simulink model "sensorMCU"  (Simulink 6.6)
settings: Solver=FixedStepDiscrete  StartTime=0.0  StopTime=10.0  FixedStep=0.01  RelTol=1e-3
InitFcn:
  | mcuInit
values from neighbouring files (symbols this model uses):
  gxGainrad = gxGain*pi/180    [mcuInit.m]
  gyGainrad = gyGain*pi/180    [mcuInit.m]
  gzGainrad = gzGain*pi/180    [mcuInit.m]
  T = 0.01    [initGPS.m]    (also in mcuInit.m)
undefined symbols (not defined in the file or in its folder): AccelParam, floatToBytes, gaind, gpsInit, gpsParse, gpsRead, gpsSeparate, gyTGain, hil_getEuler, hil_getGPSRead, hil_getRates, hil_getRawRead, hil_getVned, hil_getXYZ, hilRead, logData, loggerInit, MagParam, mzTGain, polesd, protParseDecode, protParserInit, shortToBytes, spiMasterInit, spiSend, stTGain, tmeanMz, tmeanSt, tmeanVl, u1, uartInit, uShortToBytes, vlTGain, y1, zerosd
libraries: dsPICdrivers x72, simulink x6, dspswit3 x1, dspsigops x1, xpclib x1, aerolibconvert2 x1
(part 3 of 3)

== matlab function Position-Attitude Filter/kalman filter ==
  data: bias_out output inherited; quatout output inherited; V_inertial_out output inherited; w input inherited; acc input inherited; mags input inherited; windV input inherited; dt_gps input inherited; gps_update input inherited; XY_inertial input inherited; baro input inherited; gps_psi input inherited; euler_out output inherited; pqr_out output inherited; unfiltered_euler_out output inherited; bodyAcc_out output inherited; P_out output inherited
function [bias_out, quatout,V_inertial_out,euler_out,pqr_out,unfiltered_euler_out,bodyAcc_out,P_out] = fcn(w,acc,mags,windV,dt_gps,gps_update,XY_inertial,baro,gps_psi)

    %% initialize static variables
    persistent xhat;
    persistent P;
    persistent bodyV_prev;
	persistent XY_inertial_prev;
    persistent baro_prev;
    persistent unfiltered_euler;
    persistent bodyAcc;
    persistent V_inertial;
	persistent qerr;
    persistent gps_alive;
    if isempty(xhat)
        xhat = [0.999998858349755;
                0.000871902307597;
                0.000873425393729;
                0.000871902307597;
                w+[.001;.001;.001]];
        P=diag( [ 1*ones(1,3) .05*ones(1,3) ] );
        bodyV_prev = [0;0;0];
        baro_prev = baro;
        XY_inertial_prev = [0;0];
        unfiltered_euler = [0;0;0];
        bodyAcc = [0;0;0];
        V_inertial = [0;0;0];
        qerr = [1;0;0;0];
        gps_alive = 0;
    end

    %% initialize other variables
    dt  = 0.01;      % fundamental time step
    
    B = [0.468741473405951;
         0.129010679377825;
        -0.873863648240210];
    
    Yaw_good_threshold = 6; %if GPS interpolated velocity is greater than 8, use GPS heading
    dt_gps_thresh= 2;

    H= [eye(3,3) zeros(3,3)]; % measurement matrix
    F= zeros(6,6);				% State transition matrix
    Gw=zeros(6,6);				% Noise mapping matrix
    Rw=eye(6,6);					% Process noise covariance

    % kalman filter parameters
    rwt = .02;       % error quaternion noise
    rwb = 1e-3;       % gyro bias noise
    % rwb = 0.01;
    rvv = .04;        % sensor noise
    % rvv = 0.25;

    F(1:3,4:6) = 0.5*eye(3);		% the state transition matrix
    
%     Gw(1:3,1:3) = -0.5*eye(3);	% Process Noise input
%     Gw(4:6,4:6) = eye(3);			% Process Noise input
%     Rw(1:3,1:3) = rwt^2*eye(3);	% Covariance of process noise
%     Rw(4:6,4:6) = rwb^2*eye(3);	% Covariance of process noise
%     Cd=dt*Gw*Rw*transpose(Gw);  % discreet equivalent of noise
    Cd = [diag(dt*.25*rwt^2*ones(3,1)),                   zeros(3,3);
                            zeros(3,3), diag(dt*.25*rwb^2*ones(3,1));];

	Rv = rvv^2*eye(3);			% measurement noise covariance
    
    %% integrate gyros to get new xhat
    xhat(1:4) = integ_gyros(xhat,w,dt);
    
    %% fill in the state transition matrix, Phi = expm(F*dt)
    Phi = state_transition(xhat,w,dt);
    
    %% propogate covariance: P=Phi*(P+Cd)*transpose(Phi);
    for k=1:6
        P(k,k)=P(k,k)+Cd(k,k);  % P = P+Cd
    end
    %% P=Phi*P*transpose(Phi);
    P(1:3,:)=[(Phi(1:3,1:3)*P(1:3,:)+Phi(1:3,4:6)*P(4:6,:))*transpose(Phi(1:3,:))  Phi(1:3,:)*P(:,4:6)];
    P(4:6,:)=[transpose(P(1:3,4:6)) P(4:6,4:6);];


    %% check for gps update
    if (gps_alive == 0)
        body = [0;0;0];
        [Pitch, Roll, Yaw] = accelMagsBody2euler(acc,mags,body);


        % %         q_hat = xhat(1:4);
% %         for k=1
% %             Cnb = q2dcm(q_hat);
% %             A_i = transpose(Cnb)*Gbody;
% %             B_i = transpose(Cnb)*mags;
% %             M = -[2*sk([0;0;-1]);2*sk(B)];
% %             qerr = inv(M'*M)*M'*-([A_i-[0;0;-1];B_i-B]);
% % 
% %             if norm(qerr)^2 < 1
% %                 q_hat=quatmult([sqrt(1-norm(qerr)^2);qerr],q_hat);
% %             else
% %                 q_hat=quatmult([1;qerr],q_hat);
% %             end
% %             if (q_hat(1)<0)
% %                 q_hat = -q_hat;            					% make scalar part positive
% %             end
% %           q_hat=q_hat/norm(q_hat);
% %         end

        unfiltered_euler = [Roll; Pitch; Yaw]*57.2958;
        

        
        %
        % Now use the euler angles from GPS/Acc to compute the measured quaternion
        %
        qhat = xhat(1:4);						% pull out qhat from state
        bhat = xhat(5:7);						% pull out gyro bias estimates
        qm = eul2quat([Roll Pitch Yaw]);			% measurement quaternion
        if (qm(1)<0)
            qm = -qm;            					% make scalar part positive
        end
        qerr = quatmult(quatinv(qhat),qm);			% formulate error quaternion
        if qerr(1)<0
            qerr=-qerr;
        end
%        L = P*H'*inv(H*P*H' + Rv);					% compute gains
        HPHpR = P(1:3,1:3);
        for k=1:3
            HPHpR(k,k)=HPHpR(k,k)+Rv(k,k);
        end
        invHPHpR = inv(HPHpR);
        L = P(:,1:3)*invHPHpR;					% compute gains
%        P = (eye(6) - [L zeros(6,3)])*P;						% update covariance matrix
        Mtemp = -L(1:3,:);
        for k=1:3
            Mtemp(k,k)=Mtemp(k,k)+1;
        end
        P = [                          Mtemp*P(1:3,1:3),               Mtemp*P(1:3,4:6);
             -L(4:6,:)*P(1:3,1:3)+transpose(P(1:3,4:6)),-L(4:6,:)*P(1:3,4:6)+P(4:6,4:6);];
        ds = L*qerr(2:4);								% generate updates
 %       ds = L*qerr;								% generate updates
        qhat_plus = quatmult(qhat,[1;ds(1:3)]);	% generate new attitude estimate
        bhat_plus = bhat - ds(4:6);					% generate the new gyro biases
        qhat_plus = qhat_plus/norm(qhat_plus);		% renormalize quaternion
        if (qhat_plus(1)<0)
            qhat_plus = -qhat_plus;					% make scalar part positive
        end
        xhat(1:4) = qhat_plus;				% put attitude estimate back into state
        xhat(5:7) = bhat_plus;				% put gyro bias estimates back into state

    else
%         if (gps_update)									% gps update recieved
%             if (dt_gps < dt_gps_thresh)
%                 gps_alive = 1;
%             end
%             V_inertial = ([XY_inertial-XY_inertial_prev;baro-baro_prev])/dt_gps;
%             XY_inertial_prev=XY_inertial;
%             baro_prev = baro;
%    
%             if (  (norm(V_inertial(1:2))>Yaw_good_threshold) && (gps_alive)  )
%                 Yaw = gps_psi;
%             else
%                 Yaw = quat2psi(xhat(1:4));
%             end
% 
%             Cnb = q2dcm(xhat(1:4));
%             %   aircraftV =V_inertial - windV; 				% V_gps = V_aircraft + V_wind
% 
%             bodyV=Cnb*V_inertial;
%             bodyAcc = (bodyV - bodyV_prev)/dt_gps;	% generate the body acceleration
%             if (bodyV_prev(1) == 0 && bodyV_prev(2) == 0)
%                  bodyAcc = [0;0;0];
%             end
%             bodyV_prev = bodyV;							% store body velocity for next step
% 
%             % if GPS update comes in reasonable time, use body accel, else don't
%             if gps_alive
%                  Gbody = acc - bodyAcc;
%             else
%                 Gbody = acc;
%             end
%             Gbody = Gbody/norm(Gbody)*.99999999;
%             Pitch = asin(Gbody(1));
%             Roll = asin(-Gbody(2)/cos(Pitch));
%             if sign(Gbody(3)) >= 0   % if upside down, correct phi
%                 Roll=-Roll-pi*sign(Gbody(2));
%             end
%             unfiltered_euler = [Roll; Pitch; Yaw];
%    
%             %
%             % Now use the euler angles from GPS/Acc to compute the measured quaternion
%             %
%             qhat = xhat(1:4);						% pull out qhat from state
%             bhat = xhat(5:7);						% pull out gyro bias estimates
%             qm = eul2quat([Roll Pitch Yaw]);			% measurement quaternion
%             if (qm(1)<0)
%                 qm = -qm;            					% make scalar part positive
%             end
%             qerr = quatmult(quatinv(qhat),qm);			% formulate error quaternion
%             L = P*H'*inv(H*P*H' + Rv);					% compute gains
%             P = (eye(6) - L*H)*P;						% update covariance matrix
%             ds = L*qerr(2:4);								% generate updates
%             qhat_plus = quatmult(qhat,[1;ds(1:3)]);	% generate new attitude estimate
%             bhat_plus = bhat - ds(4:6);					% generate the new gyro biases
%             qhat_plus = qhat_plus/norm(qhat_plus);		% renormalize quaternion
%             if (qhat_plus(1)<0)
%                 qhat_plus = -qhat_plus;					% make scalar part positive
%             end
%             xhat(1:4) = qhat_plus;				% put attitude estimate back into state
%             xhat(5:7) = bhat_plus;				% put gyro bias estimates back into state
%         end
    end

    
    
    P_out = P;
    quatout = xhat(1:4);
    euler_out = quat2eul(quatout);
%     euler_out = mags*pi/180;
%     euler_out = unfiltered_euler;
    euler_out(1) = -euler_out(1);
    bias_out = xhat(5:7);
    pqr_out = [w(1)-xhat(5);
               w(2)-xhat(6);
               w(3)-xhat(7);];
    unfiltered_euler_out = unfiltered_euler;
    bodyAcc_out = bodyAcc;
    V_inertial_out = V_inertial;
    
end






%================================================================
%==================   additional functions ======================
%================================================================
function quat = integ_gyros(xhat,w,dt)
    p  = w(1) - xhat(5);
    q  = w(2) - xhat(6);
    r  = w(3) - xhat(7);
    normomega    = norm([p;q;r]);
    normomegainv = inv(normomega);
    C  = cos(.5*dt*normomega);
    Sn = sin(.5*dt*normomega)*normomegainv;

    Phi_old_small = [    C, -(p *Sn), -(q* Sn), -(r *Sn);
                   (p *Sn),        C,  (r* Sn), -(q *Sn);
                   (q* Sn), -(r *Sn),        C,  (p* Sn);
                   (r* Sn),  (q *Sn), -(p* Sn),        C;];
    xhat(1:4) = Phi_old_small*xhat(1:4);	       % insert back into state
    if xhat(1)<0
        xhat(1:4)=-xhat(1:4);
    end
    quat = xhat(1:4)/norm(xhat(1:4));  %normalize quaternion
end

function Phi = state_transition(xhat,w,dt)
    p  = w(1) - xhat(5);
    q  = w(2) - xhat(6);
    r  = w(3) - xhat(7);
    p2 = p*p;
    q2 = q*q;
    r2 = r*r;
    pq = p*q;
    pr = p*r;
    qr = q*r;
    omega = sqrt(p2+q2+r2);
    omega2 = omega*omega;
    omega3 = omega2*omega;
    omega2inv = inv(omega2);
    omega3inv = inv(omega3);
    cdo = cos(dt*omega);
    sdo = sin(dt*omega);
    Phi = [       (p2 + cdo*(q2 + r2))*omega2inv, (pq - cdo*pq + omega*r*sdo)*omega2inv, (pr - cdo*pr - omega*q*sdo)*omega2inv,                 (dt*omega*p2 + (q2 + r2)*sdo)*.5*omega3inv, -(-dt*omega*pq + (-1 + cdo)*omega*r + pq*sdo)*.5*omega3inv, (dt*omega*pr + (-1 + cdo)*omega*q - pr*sdo)*.5*omega3inv;
           (pq - cdo*pq - omega*r*sdo)*omega2inv,        (q2 + cdo*(p2 + r2))*omega2inv, (qr - cdo*qr + omega*p*sdo)*omega2inv,   (dt*omega*pq + (-1 + cdo)*omega*r - pq*sdo)*.5*omega3inv,                 (dt*omega*q2 + (p2 + r2)*sdo)*.5*omega3inv,        (omega*(p - cdo*p + dt*qr) - qr*sdo)*.5*omega3inv;
           (pr - cdo*pr + omega*q*sdo)*omega2inv, (qr - cdo*qr - omega*p*sdo)*omega2inv,        (cdo*(p2 + q2) + r2)*omega2inv, -(-dt*omega*pr + (-1 + cdo)*omega*q + pr*sdo)*.5*omega3inv,       (omega*((-1 + cdo)*p + dt*qr) - qr*sdo)*.5*omega3inv,               (dt*omega*r2 + (p2 + q2)*sdo)*.5*omega3inv;
           0, 0, 0, 1, 0, 0;
           0, 0, 0, 0, 1, 0;
           0, 0, 0, 0, 0, 1];
end


function [Pitch, Roll, Yaw] = accelMagsBody2euler(acc,mags,body)
    Gbody = acc-body;
    Gbody = Gbody/norm(Gbody)*.99999999;
    Pitch = asin(Gbody(1));
    temp = -Gbody(2)/cos(Pitch);
	if abs(temp)<1
    	Roll = asin(-Gbody(2)/cos(Pitch));
	else
    	Roll = pi/2*sign(temp);
    end
        
	if sign(Gbody(3)) >= 0   % if upside down, correct phi
        Roll=-Roll-pi*sign(Gbody(2));
    end

    ct = cos(Pitch); %set up trig for less computation time
    st = sin(Pitch);
    cp = cos(Roll);
    sp = sin(Roll);
    Bflat = [ct, st*sp, cp*st;
              0,    cp,   -sp;]*mags; %rotate mags into phi=0, theta=0
	Yaw = 0.2686 -atan2g(Bflat(2),Bflat(1)); %calculate psi
end


function as=sk(a)
    % This function determines the skew-symmetric matrix
    % corresponding to a given vector a with three elements.
    	as=[0 -a(3) a(2); a(3) 0 -a(1); -a(2) a(1) 0];
end


function quat = quatmult(q1,q2)
    %   Multiplies two quaternions.
    qv1 = q1(2:4);
    qs1 = q1(1);
    qv2 = q2(2:4);
    qs2 = q2(1);

    quatv = cross(qv1,qv2) + qs1*qv2 + qs2*qv1;
    quats = qs1*qs2 - dot(qv1,qv2);

    quat = [quats;quatv];
end


function quat = quatinv(q)
    %   Inverts a quaternion.
    quat = [q(1);-q(2:4)];
end


function angles = quat2eul( q )
    qin = q./norm(q);

    y=2.*(qin(3,1).*qin(4,1) + qin(1,1).*qin(2,1));
    x=qin(1,1).^2 - qin(2,1).^2 - qin(3,1).^2 + qin(4,1).^2;
    phi = atan2g(y,x);

    theta = asin(-2.*(qin(2,1).*qin(4,1) - qin(1,1).*qin(3,1)));

    y=2.*(qin(2,1).*qin(3,1) + qin(1,1).*qin(4,1));
    x=qin(1,1).^2 + qin(2,1).^2 - qin(3,1).^2 - qin(4,1).^2;
    psi = atan2g(y,x);

    angles = [phi; theta; psi];
end


function angle = atan2g(y,x)
    angle = 0.;
    if x>0
        angle = atan(y/x);
    end
    if x==0
        angle = .5*pi*sign(y);
    end
    if x<0
        angle = pi*sign(y)+atan(y/x);
    end
end

function q = eul2quat(angles)
    % converts phi,theta,phi into q
    % lifted straight from matlab's function (with a transposed output):
    cang = cos( angles/2 );
    sang = sin( angles/2 );

    q = [ cang(:,1).*cang(:,2).*cang(:,3) + sang(:,1).*sang(:,2).*sang(:,3);
           sang(:,1).*cang(:,2).*cang(:,3) - cang(:,1).*sang(:,2).*sang(:,3);
           cang(:,1).*sang(:,2).*cang(:,3) + sang(:,1).*cang(:,2).*sang(:,3);
           cang(:,1).*cang(:,2).*sang(:,3) - sang(:,1).*sang(:,2).*cang(:,3)];
end

function dcm = q2dcm( q )
    %   The direction cosine matrix performs the coordinate
    %   transformation of a vector in inertial axes to a vector in body axes.

    qin = q; % don't need to normalize because it is already done
    %qin = quatnormalize( q );

    dcm = zeros(3,3);

    dcm(1,1) = qin(1).^2 + qin(2).^2 - qin(3).^2 - qin(4).^2;
    dcm(1,2) = 2.*(qin(2).*qin(3) + qin(1).*qin(4));
    dcm(1,3) = 2.*(qin(2).*qin(4) - qin(1).*qin(3));
    dcm(2,1) = 2.*(qin(2).*qin(3) - qin(1).*qin(4));
    dcm(2,2) = qin(1).^2 - qin(2).^2 + qin(3).^2 - qin(4).^2;
    dcm(2,3) = 2.*(qin(3).*qin(4) + qin(1).*qin(2));
    dcm(3,1) = 2.*(qin(2).*qin(4) + qin(1).*qin(3));
    dcm(3,2) = 2.*(qin(3).*qin(4) - qin(1).*qin(2));
    dcm(3,3) = qin(1).^2 - qin(2).^2 - qin(3).^2 + qin(4).^2;
end



% function Cd=disrw(F,G,Ts,Rwpsd)
% %----------------------------------------------------------------
% %   function [Cd]=disrw(F,G,T,Rwpsd)
% %
% %   disrw computes the discrete equivalent of continous noise for the
% %   dynamic system described by
% %
% %                            x_dot = Fx + Gw
% %
% %   w is the driving noise.  Ts is the sampling time and Rwpsd
% %   is the power spectral density of the driving noise.
% %
% %---------------------------------------------------------------------
% 
% ZF=zeros(size(F));
% [n,m]=size(G);
% ME=[-F G*Rwpsd*G';
%     ZF F'];
% phi=expm(ME*Ts);
% phi12=phi(1:n,n+1:2*n);
% phi22=phi(n+1:2*n,n+1:2*n);
% Cd=phi22'*phi12;
% 
% end

== matlab function myMux Fun4 ==
  data: u1 input inherited; y output inherited; u2 input inherited
function y = myMux(u1, u2)
% This block supports an embeddable subset of the MATLAB language.
% See the help menu for details. 

y = [u1(1:12); u2(1:12)];

== matlab function myMux Fun1 ==
  data: u1 input inherited; y output inherited; u2 input inherited; u3 input inherited
function y = myMux(u1, u2, u3)
% This block supports an embeddable subset of the MATLAB language.
% See the help menu for details. 

y = zeros(3,1);
y(1) = u1(1);
y(2) = u2(1);
y(3) = u3(1);

== matlab function Position-Attitude Filter/myMux Fun4 ==
  data: u1 input inherited; y output inherited; u2 input inherited
function y = myMux(u1, u2)
% This block supports an embeddable subset of the MATLAB language.
% See the help menu for details. 

y = [u1(1:2); u2];

== matlab function Sensor Data/Raw Sensors/Sensor Suite/myMux Fun3 ==
  data: u1 input inherited; y output inherited; u2 input inherited; u3 input inherited
function y = myMux(u1, u2, u3)
% This block supports an embeddable subset of the MATLAB language.
% See the help menu for details. 

y = [u1(1); u2(1); u3(1)];

== matlab function Sensor Data/Raw Sensors/Sensor Suite/Calibration and Temperature Compensation/Enables/Disables the Computation of initial Biases and Temps ==
  data: tOut output inherited
function tOut = getTIni

persistent aveCount;
persistent tIni;

if isempty(aveCount)
    aveCount =1;
    tIni = 1;
end;

if aveCount < 500
    aveCount = aveCount + 1;
end

if aveCount == 500
    tIni =0;
    aveCount = aveCount + 1;
end

tOut = tIni;

%if aveCount > 500
%    tIni = 0;
%end

% if isempty(aveCount)
%     aveCount =1;
%     initBias = [0.0 0.0 0.0]';
% end;
%     
% if (aveCount<10)
%     initBias = initBias+ Raw;
%     bias = initBias/aveCount;
%     aveCount = aveCount +1;
% end;
% 
% if (aveCount == 10)
%     initBias = initBias/(aveCount-1);
%     aveCount = 100;
% end;
% 
% if (aveCount == 100)
%     bias = initBias;
% end;

== matlab function Sensor Data/Load Msg/myMux Fun ==
  data: u1 input inherited; y output inherited; u2 input inherited; u3 input inherited
function y = myMux(u1, u2, u3)
% This block supports an embeddable subset of the MATLAB language.
% See the help menu for details. 

y = [u1; u2; u3(1); u3(2)];

== matlab function Sensor Data/Raw Sensors/Sensor Suite/Magnetometer Driver and Low Pass/myMux Fun1 ==
  data: u1 input inherited; y output inherited; u2 input inherited; u3 input inherited
function y = myMux(u1, u2, u3)
% This block supports an embeddable subset of the MATLAB language.
% See the help menu for details. 

y = [u1(1); u2(1); u3(1)];

== matlab function Sensor Data/Raw Sensors/Sensor Suite/myMux Fun1 ==
  data: u1 input inherited; y output inherited; u2 input inherited; u3 input inherited
function y = myMux(u1, u2, u3)
% This block supports an embeddable subset of the MATLAB language.
% See the help menu for details. 

y = [u1(1); u2(1); u3(1)];

== matlab function Sensor Data/Raw Sensors/Sensor Suite/myMux Fun2 ==
  data: u1 input inherited; y output inherited; u2 input inherited; u3 input inherited
function y = myMux(u1, u2, u3)
% This block supports an embeddable subset of the MATLAB language.
% See the help menu for details. 

y = [u1(1); u2(1); u3(1)];

== matlab function Sensor Data/Raw Sensors/myMux Fun ==
  data: u1 input inherited; y output inherited; u2 input inherited; u3 input inherited
function y = myMux(u1, u2, u3)
% This block supports an embeddable subset of the MATLAB language.
% See the help menu for details. 

y = [u1(:); u2(:); u3(:)];

== matlab function Diagnostic Data/myMux Fun2 ==
  data: u1 input inherited; y output inherited; u2 input inherited; u3 input inherited; u4 input inherited
function y = myMux(u1, u2, u3, u4)
% This block supports an embeddable subset of the MATLAB language.
% See the help menu for details. 


y = [u1(:); u2; u3; u4];

== matlab function myMux Fun2 ==
  data: u1 input inherited; y output inherited; u2 input inherited; u3 input inherited
function y = myMux(u1, u2, u3)
% This block supports an embeddable subset of the MATLAB language.
% See the help menu for details. 

y = [u1(1:12); u2(1:12); u3(1:2)];

== matlab function Sensor Data/Raw Sensors/Sensor Suite/Subsystem/myMux Fun3 ==
  data: u1 input inherited; y output inherited; u2 input inherited
function y = myMux(u1, u2)
% This block supports an embeddable subset of the MATLAB language.
% See the help menu for details. 

y = [u1(1); u2(1)];

== matlab function myMux Fun3 ==
  data: u1 input inherited; y output inherited; u2 input inherited
function y = myMux(u1, u2)
% This block supports an embeddable subset of the MATLAB language.
% See the help menu for details. 

y = [u1(1:12); u2(1:12)];

== matlab function Sensor Data/Raw Sensors/Sensor Suite/Calibration and Temperature Compensation/Initial Bias and Temp/myMux Fun1 ==
  data: u1 input inherited; y output inherited; u2 input inherited; u3 input inherited
function y = myMux(u1, u2, u3)
% This block supports an embeddable subset of the MATLAB language.
% See the help menu for details. 

y = [u1(1); u2(1); u3(1)];

== matlab function Control Surface Input/myMux Fun5 ==
  data: u1 input inherited; y output inherited; u2 input inherited; u3 input inherited; u4 input inherited; u5 input inherited
function y = myMux(u1, u2, u3, u4, u5)
% This block supports an embeddable subset of the MATLAB language.
% See the help menu for details. 

y = uint8(zeros(10,1));
y(1) = u1(1);
y(2) = u1(2);
y(3) = u2(1);
y(4) = u2(2);
y(5) = u3(1);
y(6) = u3(2);
y(7) = u4(1);
y(8) = u4(2);
y(9) = u5(1);
y(10) = u5(2);
